simulink library "Gravity_UL"  (R2019a)
settings: Solver=VariableStepAuto  StartTime=0.0  StopTime=10.0  RelTol=1e-3
undefined symbols (not defined in the file): ENV, Motor, VEH
libraries: simulink x2
settings Model: Creator=John Jr  LastModifiedBy=John Jr

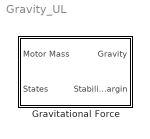
== system Gravity_UL ==
  Gravitational Force : Subsystem  mask{g=ENV.g, m=VEH.m, CG1=VEH.CG_1, CG2=VEH.CG_2, CP=VEH.CP, t_b=Motor.t_b}
      mask prompts: g "Gravitational acceleration [m/s^2]"; m "Vehicle mass without motor [kg]"; CG1 "CG on launchpad [m]"; CG2 "CG after motor burn [m]"; CP "Center of pressure [m]"; t_b "Total motor burn time [s]"
      mask DialogControl DescGroupVar Prompt: Gravitational Force Library
      mask DialogControl DescTextVar Prompt: This block models the gravitational force acting on the vehicle, as well as the stability margin as the motor burns.
      mask DialogControl Control2 Prompt: Stability Properties (measured from nosecone):
      mask Display:
      | patch([0 1 1 0], [0 0 1 1],[.8 1 1])
      | 
      | port_label('input',1,'\fontname{Cambria Math}M_{motor} [kg]','texmode','on')
      | port_label('input',2,'\fontname{Cambria Math}States','texmode','on')
      | 
      | port_label('output',1,'\fontname{Cambria Math}Gravity [N]','texmode','on')
      | port_label('output',2,'\fontname{Cambria Math}CG-CP [m]','texmode','on')

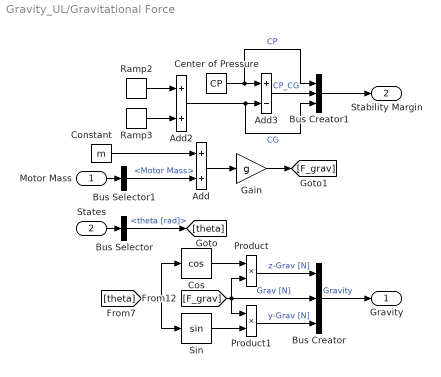
== system Gravity_UL/Gravitational Force ==
  Motor Mass : Inport
  States : Inport  Port=2
  Add : Sum
  Add2 : Sum
  Add3 : Sum  Inputs=+-
  Bus Creator : BusCreator  Inputs=3
  Bus Creator1 : BusCreator  Inputs=3
  Bus Selector : BusSelector  OutputSignals=theta.theta [rad]
  Bus Selector1 : BusSelector  OutputSignals=Motor Mass
  Center of Pressure : Constant  Value=CP
  Constant : Constant  Value=m
  Cos : Trigonometry  Operator=cos
  Gain : Gain  Gain=g
  Product : Product
  Product1 : Product
  Ramp2 : simulink/Sources/Ramp  slope=-(CG1-CG2)/t_b  start=0  InitialOutput=CG1
  Ramp3 : simulink/Sources/Ramp  slope=(CG1-CG2)/t_b  start=t_b  InitialOutput=0
  Sin : Trigonometry
  Gravity : Outport
  Stability Margin : Outport  Port=2
  wires:
  Bus Selector/1 -> [theta]  "<theta [rad]>"
  Bus Selector1/1 -> Add/2  "<Motor Mass>"
  Motor Mass/1 -> Bus Selector1/1
  States/1 -> Bus Selector/1
  Add/1 -> Gain/1
  Constant/1 -> Add/1
  Ramp3/1 -> Add2/2
  Ramp2/1 -> Add2/1
  Center of Pressure/1 -> Bus Creator1/1, Add3/1  "CP"
  Add2/1 -> Bus Creator1/3, Add3/2  "CG"
  [F_grav] -> Bus Creator/2, Product1/1, Product/2  "Grav [N]"
  Gain/1 -> [F_grav]
  Cos/1 -> Product/1
  Sin/1 -> Product1/2
  [theta] -> Sin/1, Cos/1
  Product1/1 -> Bus Creator/3  "y-Grav [N]"
  Product/1 -> Bus Creator/1  "z-Grav [N]"
  Bus Creator/1 -> Gravity/1  "Gravity"
  Bus Creator1/1 -> Stability Margin/1
  Add3/1 -> Bus Creator1/2  "CP_CG"
